simulink model "UAVUGVMatlabFunction"  (R2018a)
settings: Solver=VariableStepAuto  StartTime=0.0  StopTime=10.0  RelTol=1e-3
libraries: simulink x1
settings Model: Creator=wangluo  LastModifiedBy=wangluo

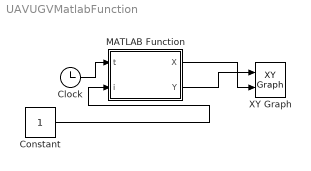
== system UAVUGVMatlabFunction ==
  Clock : Clock
      settings: Decimation=100
  Constant : Constant
  MATLAB Function : MATLAB Function  TreatAsAtomicUnit=on
  XY Graph : simulink/Sinks/XY Graph  xmin=-1  xmax=1  ymin=-1  ymax=1  st=-1
  wires:
  MATLAB Function/1(X) -> XY Graph/2
  MATLAB Function/2(Y) -> XY Graph/1
  Clock/1 -> MATLAB Function/1(t)
  Constant/1 -> MATLAB Function/2(i)

== matlab function UAVUGVMatlabFunction/MATLAB Function ==
  data: t input; X output; Y output; i input
function [X, Y] = fcn(t,i)
% #codegen
X = -8;
Y = -8;
X(:,i) = -8;
Y(:,i) = -8;

if (0<=t)&&(t<=30)
    i = i+1;  %j = j+1;
    speed = 1;
    theta = 0;
%     X(:,i) = X(:,i-1) + speed * t * cos(pi/180 * theta);
    X(:,i) = 9;
    Y = Y + speed * t * sin(pi/180 * theta);
    
end
if (30<=t)&&(t<=60)
    i = i+1;  %j = j+1;
    speed = 1;
    theta = 90;
    X = X + speed * (t-30) * cos(pi/180 * theta);
    Y = Y + speed * (t-30) * sin(pi/180 * theta);
end
